simulink model "Simulation-SmartRefrigerator"  (R2019a)
settings: Solver=VariableStepAuto  StartTime=0.0  StopTime=10.0  RelTol=1e-3
settings Model: Creator=shivam  LastModifiedBy=shivam

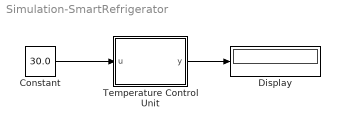
== system Simulation-SmartRefrigerator ==
  Constant : Constant  Value=30.0
  Display : Display
  Temperature Control Unit : MATLAB Function  TreatAsAtomicUnit=on
  wires:
  Constant/1 -> Temperature Control Unit/1(u)
  Temperature Control Unit/1(y) -> Display/1

== matlab function Simulation-SmartRefrigerator/Temperature Control Unit ==
  data: u input; y output
function y = fcn(u)
    if u >= 35.0
        y = 5;
    end
    if u >= 32.5 && u < 35.0
        y = 4;
    end
    if u >= 30.0 && u < 32.5
        y = 3;
    end
    if u >= 25.0 && u < 30.0
        y = 2;
    end
    if u >= 20.0 && u < 25.0
        y = 1;
    end
    if u < 5.0
        y = 5;
    end
